simulink model "ControlObsSemCanal2011"  (Simulink 7.7)
settings: Solver=ode45  SolverMode=SingleTasking  StartTime=0.0  StopTime=20.0  RelTol=1e-3
values from neighbouring files (symbols this model uses):
  C = GYzss.C    [ProjetoControlPI.m]    (also in ident.m)
  F = FKi(1:size(G,2))    [ProjetoControlPI.m]    (also in ident.m = acker(G, H, P))
  G = GYzss.A    [ProjetoControlPI.m]    (also in ident.m)
  H = GYzss.B    [ProjetoControlPI.m]    (also in ident.m)
  Kc = 1/Y(end)    [ProjetoControlPI.m]    (also in ident.m = dcgain(SysCtl))
  L = L'    [ProjetoControlPI.m]    (also in ident.m)
libraries: simulink x2
settings Model: Creator=castr  LastModifiedBy=castr  CovMetricSettings=dwe  CovHtmlReporting=off  covSaveCumulativeToWorkspaceVar=off  CovSaveSingleToWorkspaceVar=off  CovExternalEMLEnable=on
settings DataIOCC: LimitDataPoints=off  SaveFormat=StructureWithTime  SignalLoggingSaveFormat=Dataset
settings OptimizationCC: ExpressionDepthLimit=128
settings DebuggingCC: UnderspecifiedInitializationDetection=Simplified  MergeDetectMultiDrivingBlocksExec=error  SolverPrmCheckMsg=none  FcnCallInpInsideContextMsg=Enable All  StateNameClashWarn=none  SFUnexpectedBacktrackingDiag=error  SFNoUnconditionalDefaultTransitionDiag=error
settings HardwareCC: ProdBitPerPointer=64  ProdLargestAtomicFloat=Float  ProdIntDivRoundTo=Zero  ProdEndianess=LittleEndian  ProdHWDeviceType=Specified
settings CodeAppCC: CustomSymbolStrType=$N$R$M_T
settings GRTTargetCC: TargetFunctionLibrary=C99 (ISO)  GeneratePreprocessorConditionals=Use local settings

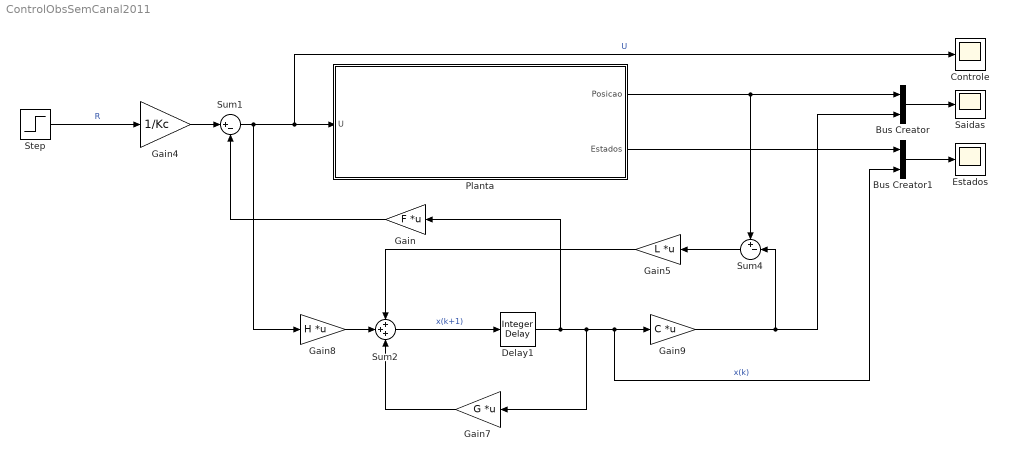
== system ControlObsSemCanal2011 ==
  Bus Creator : BusCreator  Inputs=2
  Bus Creator1 : BusCreator  Inputs=2
  Controle : Scope
      settings: TimeRange=auto  MaxDataPoints=5000  SaveToWorkspace=off  SaveName=ScopeData2  YMin=-1.28663  YMax=3.43728  SampleTime=-1
  Delay1 : simulink/Discrete/Integer Delay  NumDelays=1  vinit=0.0  samptime=Ts
  Estados : Scope
      settings: TimeRange=auto  MaxDataPoints=5000  SaveToWorkspace=off  YMin=-13.81568  YMax=8.75377  SampleTime=-1
  Gain : Gain  Gain=F  Multiplication=Matrix(K*u)
  Gain4 : Gain  Gain=1/Kc
  Gain5 : Gain  Gain=L  Multiplication=Matrix(K*u)
  Gain7 : Gain  Gain=G  Multiplication=Matrix(K*u)
  Gain8 : Gain  Gain=H  Multiplication=Matrix(K*u)
  Gain9 : Gain  Gain=C  Multiplication=Matrix(K*u)
  Planta : Subsystem
  Saidas : Scope
      settings: TimeRange=auto  MaxDataPoints=5000  SaveToWorkspace=off  SaveName=ScopeData  YMin=-0.64688  YMax=1.83714  SampleTime=-1
  Step : Step  SampleTime=0
  Sum1 : Sum  Inputs=|+-
  Sum2 : Sum  Inputs=+++
  Sum4 : Sum  Inputs=+-|
  wires:
  Sum1/1 -> Gain8/1, Controle/1, Planta/1(U)  "U"
  Gain/1 -> Sum1/2
  Step/1 -> Gain4/1  "R"
  Bus Creator/1 -> Saidas/1
  Sum2/1 -> Delay1/1  "x(k+1)"
  Delay1/1 -> Gain/1, Gain9/1, Bus Creator1/2, Gain7/1  "x(k)"
  Gain4/1 -> Sum1/1
  Gain9/1 -> Sum4/2, Bus Creator/2
  Sum4/1 -> Gain5/1
  Gain7/1 -> Sum2/3
  Gain8/1 -> Sum2/2
  Gain5/1 -> Sum2/1
  Planta/1(Posicao) -> Sum4/1, Bus Creator/1
  Bus Creator1/1 -> Estados/1
  Planta/2(Estados) -> Bus Creator1/1

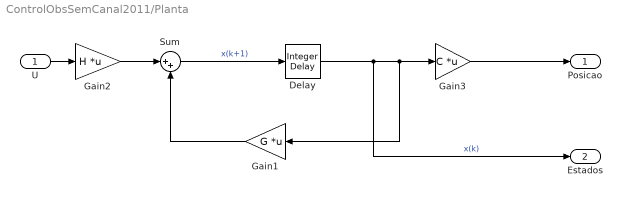
== system ControlObsSemCanal2011/Planta ==
  U : Inport
  Delay : simulink/Discrete/Integer Delay  NumDelays=1  vinit=[0 0]  samptime=Ts
  Gain1 : Gain  Gain=G  Multiplication=Matrix(K*u)
  Gain2 : Gain  Gain=H  Multiplication=Matrix(K*u)
  Gain3 : Gain  Gain=C  Multiplication=Matrix(K*u)
  Sum : Sum  Inputs=|++
  Posicao : Outport
  Estados : Outport  Port=2
  wires:
  Gain1/1 -> Sum/2
  Gain2/1 -> Sum/1
  U/1 -> Gain2/1
  Sum/1 -> Delay/1  "x(k+1)"
  Delay/1 -> Estados/1, Gain1/1, Gain3/1  "x(k)"
  Gain3/1 -> Posicao/1
